simulink model "untitled"  (R2014b)
settings: Solver=ode45  StartTime=0.0  StopTime=10.0  RelTol=1e-3
settings Model: Creator=rajab  LastModifiedBy=rajab

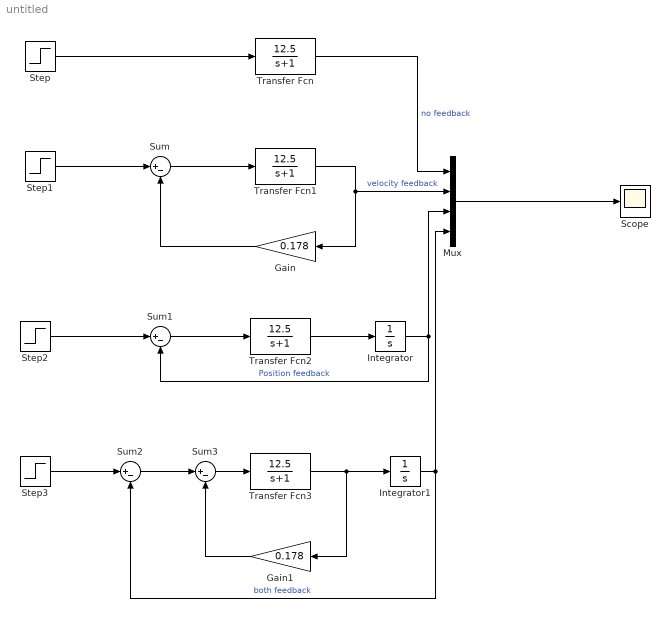
== system untitled ==
  Gain : Gain  Gain=0.178
  Gain1 : Gain  Gain=0.178
  Integrator : Integrator
  Integrator1 : Integrator
  Mux : Mux
  Scope : Scope
      settings: ShowLegends=on
  Step{,1..3} (4 alike) : Step  SampleTime=0
  Sum{,1..3} (4 alike) : Sum  Inputs=|+-
  Transfer Fcn{,1..3} (4 alike) : TransferFcn  Numerator=[12.5]  Denominator=[1 1]
  wires:
  Mux/1 -> Scope/1
  Step/1 -> Transfer Fcn/1
  Step1/1 -> Sum/1
  Sum/1 -> Transfer Fcn1/1
  Step2/1 -> Sum1/1
  Sum1/1 -> Transfer Fcn2/1
  Transfer Fcn2/1 -> Integrator/1
  Step3/1 -> Sum2/1
  Sum2/1 -> Sum3/1
  Sum3/1 -> Transfer Fcn3/1
  Transfer Fcn3/1 -> Gain1/1, Integrator1/1
  Transfer Fcn1/1 -> Gain/1, Mux/2  "velocity feedback"
  Gain/1 -> Sum/2
  Transfer Fcn/1 -> Mux/1  "no feedback"
  Integrator/1 -> Sum1/2, Mux/3  "Position feedback"
  Integrator1/1 -> Mux/4, Sum2/2  "both feedback"
  Gain1/1 -> Sum3/2
